simulink model "Task3"  (R2021a)
settings: Solver=FixedStepDiscrete  StartTime=0.0  StopTime=10.0  RelTol=1e-3  EnableMultiTasking=on
settings Model: Creator=Alaa  LastModifiedBy=Alaa
settings DataIOCC: ReturnWorkspaceOutputs=off
settings OptimizationCC: DefaultParameterBehavior=Inlined  InlineInvariantSignals=on  EnableMemcpy=off  LifeSpan=1  EfficientTunableParamExpr=on
settings DebuggingCC: UnderspecifiedInitializationDetection=Classic  MergeDetectMultiDrivingBlocksExec=none  SFMachineParentedDataDiag=warning  ArithmeticOperatorsInVariantConditions=warning
settings ModelReferenceCC: PropagateSignalLabelsOutOfModel=off
settings SFSimCC: MATLABDynamicMemAlloc=off  CustomCodeUndefinedFunction=UseInterfaceOnly
settings RTWCC: SystemTargetFile=ert.tlc  GenCodeOnly=on  TemplateMakefile=ert_default_tmf  GenerateReport=on  IncludeHyperlinkInReport=on  LaunchReport=on  GenerateTraceInfo=on  GenerateTraceReport=on  GenerateTraceReportSl=on  GenerateTraceReportSf=on  GenerateTraceReportEml=on
settings CodeAppCC: ForceParamTrailComments=on  IgnoreCustomStorageClasses=off  OperatorAnnotations=on  SimulinkDataObjDesc=on  SFDataObjDesc=on  MATLABFcnDesc=on  InsertBlockDesc=on  StateflowObjectComments=on  MATLABSourceComments=on
settings ERTTargetCC: MultiwordLength=2048  GenerateSampleERTMain=on  InlinedParameterPlacement=NonHierarchical  ERTCustomFileTemplate=example_file_process.tlc

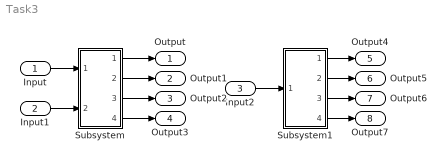
== system Task3 ==
  Input : Inport
  Input1 : Inport  Port=2
  Input2 : Inport  Port=3
  Subsystem : Subsystem
  Subsystem1 : Subsystem
  Output : Outport
  Output1 : Outport  Port=2
  Output2 : Outport  Port=3
  Output3 : Outport  Port=4
  Output4 : Outport  Port=5
  Output5 : Outport  Port=6
  Output6 : Outport  Port=7
  Output7 : Outport  Port=8
  wires:
  Input/1 -> Subsystem/1(In1)
  Input1/1 -> Subsystem/2(In2)
  Subsystem/1(Out1) -> Output/1
  Subsystem/2(Out2) -> Output1/1
  Subsystem/3(Out3) -> Output2/1
  Subsystem/4(Out4) -> Output3/1
  Input2/1 -> Subsystem1/1(In1)
  Subsystem1/1(Out1) -> Output4/1
  Subsystem1/2(Out2) -> Output5/1
  Subsystem1/3(Out3) -> Output6/1
  Subsystem1/4(Out4) -> Output7/1

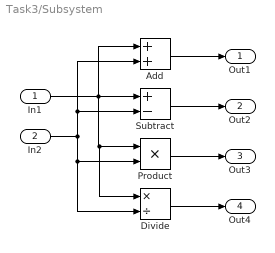
== system Task3/Subsystem ==
  In1 : Inport
  In2 : Inport  Port=2
  Add : Sum
  Divide : Product  Inputs=*/
  Product : Product
  Subtract : Sum  Inputs=+-
  Out1 : Outport
  Out2 : Outport  Port=2
  Out3 : Outport  Port=3
  Out4 : Outport  Port=4
  wires:
  In1/1 -> Add/1, Divide/1, Product/1, Subtract/1
  In2/1 -> Add/2, Subtract/2, Divide/2, Product/2
  Divide/1 -> Out4/1
  Product/1 -> Out3/1
  Subtract/1 -> Out2/1
  Add/1 -> Out1/1

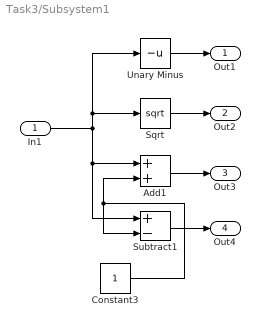
== system Task3/Subsystem1 ==
  In1 : Inport
  Add1 : Sum
  Constant3 : Constant
  Sqrt : Sqrt  SaturateOnIntegerOverflow=on
  Subtract1 : Sum  Inputs=+-
  Unary Minus : UnaryMinus  SaturateOnIntegerOverflow=on
  Out1 : Outport
  Out2 : Outport  Port=2
  Out3 : Outport  Port=3
  Out4 : Outport  Port=4
  wires:
  In1/1 -> Subtract1/1, Add1/1, Unary Minus/1, Sqrt/1
  Add1/1 -> Out3/1
  Constant3/1 -> Add1/2, Subtract1/2
  Subtract1/1 -> Out4/1
  Unary Minus/1 -> Out1/1
  Sqrt/1 -> Out2/1
